simulink model "Lab1_Nonlinear"  (R2020b)
settings: Solver=VariableStepAuto  StartTime=0.0  StopTime=100  RelTol=1e-3
values from neighbouring files (symbols this model uses):
  a = 24    [Lab1.m]
  gHFast = inv(1*inv(0 + 1*kHFast)*1)    [Lab1.m]
  gThetaFast = inv(1*inv(0 + 1*kThetaFast)*1)    [Lab1.m]
  H0 = 16    [Lab1.m]
  kHFast = Fe(1)    [Lab1.m]
  kThetaFast = Fe(1)    [Lab1.m]
  Q0 = 48    [Lab1.m]
  S = pi*5*5    (= 78.5398163397)    [Lab1.m]
  T0 = 45    [Lab1.m]
  Tc = 20    [Lab1.m]
  Tw = 70    [Lab1.m]
settings Model: Creator=DELL  LastModifiedBy=DELL

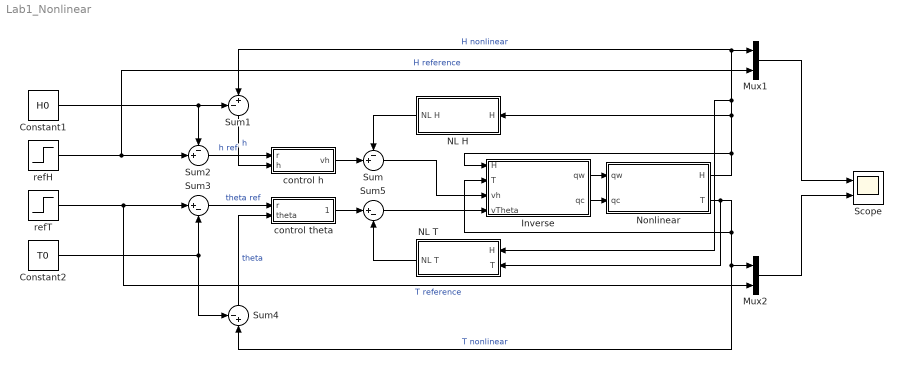
== system Lab1_Nonlinear ==
  Constant1 : Constant  Value=H0
  Constant2 : Constant  Value=T0
  Inverse : Subsystem
  Mux1 : Mux  Inputs=2
  Mux2 : Mux  Inputs=2
  NL H : Subsystem
  NL T : Subsystem
  Nonlinear : Subsystem
  Scope : Scope  NumInputPorts=2
  Sum{,1..2,4} (4 alike) : Sum  Inputs=-+|
  Sum3 : Sum  Inputs=|+-
  Sum5 : Sum  Inputs=|+-
  control h : Subsystem
  control theta : Subsystem
  refH : Step  Before=H0  After=20  SampleTime=0
  refT : Step  Before=T0  After=50  SampleTime=0
  wires:
  Nonlinear/2(T) -> Inverse/2(T), Sum4/2, Mux2/1, NL T/2(T)  "T nonlinear"
  Sum3/1 -> control theta/1(r)  "theta ref"
  Inverse/2(qc) -> Nonlinear/2(qc)
  Sum2/1 -> control h/1(r)  "h ref"
  refH/1 -> Sum2/2, Mux1/2  "H reference"
  Inverse/1(qw) -> Nonlinear/1(qw)
  Nonlinear/1(H) -> NL H/1(H), Sum1/2, Mux1/1, NL T/1(H), Inverse/1(H)  "H nonlinear"
  refT/1 -> Mux2/2, Sum3/1  "T reference"
  Mux1/1 -> Scope/1
  Constant2/1 -> Sum4/1, Sum3/2
  Mux2/1 -> Scope/2
  Constant1/1 -> Sum1/1, Sum2/1
  Sum1/1 -> control h/2(h)  "h"
  Sum4/1 -> control theta/2(theta)  "theta"
  control h/1(vh) -> Sum/2
  Sum/1 -> Inverse/3(vh)
  control theta/1(vTheta) -> Sum5/1
  NL T/1(NL T) -> Sum5/2
  NL H/1(NL H) -> Sum/1
  Sum5/1 -> Inverse/4(vTheta)

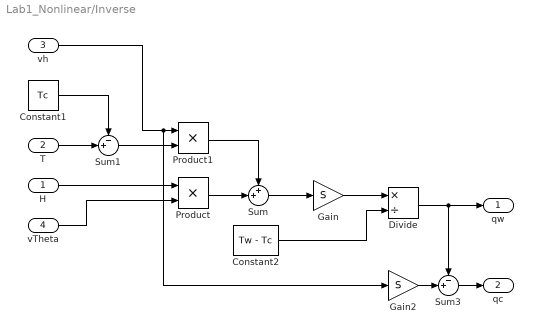
== system Lab1_Nonlinear/Inverse ==
  H : Inport
  T : Inport  Port=2
  vh : Inport  Port=3
  vTheta : Inport  Port=4
  Constant1 : Constant  Value=Tc
  Constant2 : Constant  Value=Tw - Tc
  Divide : Product  Inputs=*/
  Gain : Gain  Gain=S
  Gain2 : Gain  Gain=S
  Product : Product
  Product1 : Product
  Sum : Sum  Inputs=++|
  Sum1 : Sum  Inputs=-+|
  Sum3 : Sum  Inputs=-+|
  qw : Outport
  qc : Outport  Port=2
  wires:
  vTheta/1 -> Product/2
  H/1 -> Product/1
  T/1 -> Sum1/2
  Constant1/1 -> Sum1/1
  Sum1/1 -> Product1/2
  vh/1 -> Gain2/1, Product1/1
  Product/1 -> Sum/2
  Product1/1 -> Sum/1
  Sum/1 -> Gain/1
  Gain/1 -> Divide/1
  Constant2/1 -> Divide/2
  Divide/1 -> Sum3/1, qw/1
  Gain2/1 -> Sum3/2
  Sum3/1 -> qc/1

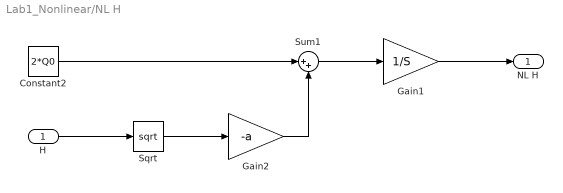
== system Lab1_Nonlinear/NL H ==
  H : Inport
  Constant2 : Constant  Value=2*Q0
  Gain1 : Gain  Gain=1/S
  Gain2 : Gain  Gain=-a
  Sqrt : Sqrt  SaturateOnIntegerOverflow=on
  Sum1 : Sum  Inputs=|++
  NL H : Outport
  wires:
  Constant2/1 -> Sum1/1
  Gain1/1 -> NL H/1
  H/1 -> Sqrt/1
  Sqrt/1 -> Gain2/1
  Gain2/1 -> Sum1/2
  Sum1/1 -> Gain1/1

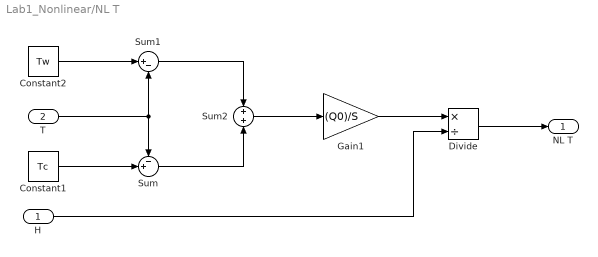
== system Lab1_Nonlinear/NL T ==
  H : Inport
  T : Inport  Port=2
  Constant1 : Constant  Value=Tc
  Constant2 : Constant  Value=Tw
  Divide : Product  Inputs=*/
  Gain1 : Gain  Gain=(Q0)/S
  Sum : Sum  Inputs=-+|
  Sum1 : Sum  Inputs=|+-
  Sum2 : Sum  Inputs=+|+
  NL T : Outport
  wires:
  Constant2/1 -> Sum1/1
  T/1 -> Sum/1, Sum1/2
  Constant1/1 -> Sum/2
  Sum1/1 -> Sum2/1
  Sum/1 -> Sum2/2
  Sum2/1 -> Gain1/1
  Gain1/1 -> Divide/1
  H/1 -> Divide/2
  Divide/1 -> NL T/1

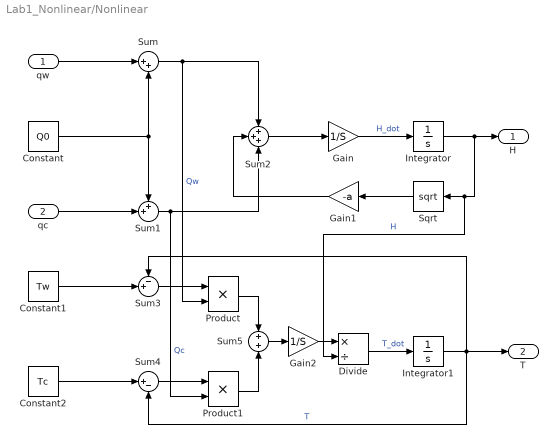
== system Lab1_Nonlinear/Nonlinear ==
  qw : Inport
  qc : Inport  Port=2
  Constant : Constant  Value=Q0
  Constant1 : Constant  Value=Tw
  Constant2 : Constant  Value=Tc
  Divide : Product  Inputs=*/
  Gain : Gain  Gain=1/S
  Gain1 : Gain  Gain=-a
  Gain2 : Gain  Gain=1/S
  Integrator : Integrator  InitialCondition=H0
  Integrator1 : Integrator  InitialCondition=T0
  Product : Product
  Product1 : Product
  Sqrt : Sqrt  SaturateOnIntegerOverflow=on
  Sum : Sum  Inputs=|++
  Sum1 : Sum  Inputs=++|
  Sum2 : Sum  Inputs=+++
  Sum3 : Sum  Inputs=-+|
  Sum4 : Sum  Inputs=|+-
  Sum5 : Sum  Inputs=+|+
  H : Outport
  T : Outport  Port=2
  wires:
  qw/1 -> Sum/1
  Constant/1 -> Sum/2, Sum1/1
  qc/1 -> Sum1/2
  Sum/1 -> Product/2, Sum2/1  "Qw"
  Sum1/1 -> Product1/2, Sum2/3  "Qc"
  Integrator/1 -> Divide/2, Sqrt/1, H/1  "H"
  Sum2/1 -> Gain/1
  Gain/1 -> Integrator/1  "H_dot"
  Gain1/1 -> Sum2/2
  Sqrt/1 -> Gain1/1
  Integrator1/1 -> Sum4/2, T/1, Sum3/1  "T"
  Constant2/1 -> Sum4/1
  Constant1/1 -> Sum3/2
  Sum3/1 -> Product/1
  Sum4/1 -> Product1/1
  Sum5/1 -> Gain2/1
  Product/1 -> Sum5/1
  Product1/1 -> Sum5/2
  Gain2/1 -> Divide/1
  Divide/1 -> Integrator1/1  "T_dot"

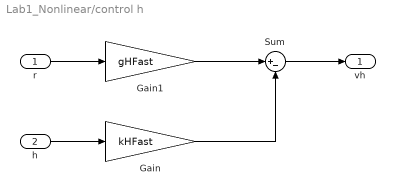
== system Lab1_Nonlinear/control h ==
  r : Inport
  h : Inport  Port=2
  Gain : Gain  Gain=kHFast
  Gain1 : Gain  Gain=gHFast
  Sum : Sum  Inputs=|+-
  vh : Outport
  wires:
  r/1 -> Gain1/1
  h/1 -> Gain/1
  Gain1/1 -> Sum/1
  Gain/1 -> Sum/2
  Sum/1 -> vh/1

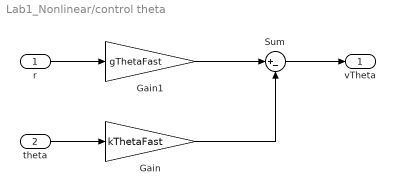
== system Lab1_Nonlinear/control theta ==
  r : Inport
  theta : Inport  Port=2
  Gain : Gain  Gain=kThetaFast
  Gain1 : Gain  Gain=gThetaFast
  Sum : Sum  Inputs=|+-
  vTheta : Outport
  wires:
  r/1 -> Gain1/1
  theta/1 -> Gain/1
  Gain1/1 -> Sum/1
  Gain/1 -> Sum/2
  Sum/1 -> vTheta/1
